simulink model "SecRwRtStFtrstHolderChk"  (R2018b)
settings: Solver=FixedStepDiscrete  StartTime=0.0  StopTime=10.0  FixedStep=0.01  RelTol=1e-3
libraries: simulink x1
settings Model: ModifiedHistory=2023/11/7Bug 555794 童锁需要停止 21-26  Creator=sn2xws  LastModifiedBy=sn2xws
settings DataIOCC: SaveFormat=StructureWithTime
settings OptimizationCC: DefaultParameterBehavior=Inlined  EnhancedBackFolding=on  PassReuseOutputArgsAs=Individual arguments  ZeroExternalMemoryAtStartup=off  ZeroInternalMemoryAtStartup=off  OptimizeBlockOrder=speed  DifferentSizesBufferReuse=on  OptimizationCustomize=off
settings DebuggingCC: ParameterTunabilityLossMsg=error
settings ModelReferenceCC: ModelReferenceNumInstancesAllowed=Single
settings SFSimCC: MATLABDynamicMemAlloc=off
settings RTWCC: SystemTargetFile=autosar.tlc  GenCodeOnly=on  TemplateMakefile=ert_default_tmf  Description=AUTOSAR  GenerateReport=on  IncludeHyperlinkInReport=on  LaunchReport=on  GenerateTraceInfo=on  GenerateTraceReport=on  GenerateTraceReportSl=on  GenerateTraceReportSf=on  GenerateTraceReportEml=on
settings CodeAppCC: ForceParamTrailComments=on  IgnoreCustomStorageClasses=off  OperatorAnnotations=on  SimulinkDataObjDesc=on  SFDataObjDesc=on  InsertBlockDesc=on
settings STFCustomTargetCC: TargetLangStandard=C99 (ISO)  MultiwordLength=256  ParMdlRefBuildCompliant=on  CompOptLevelCompliant=on  IncludeMdlTerminateFcn=off  CombineOutputUpdateFcns=on  SuppressErrorStatus=on  ERTCustomFileBanners=on  SupportNonFinite=off  SupportComplex=off  SupportContinuousTime=off  SupportNonInlinedSFcns=off  RemoveResetFunc=on  MATLABClassNameForMDSCustomization=Simulink.SoftwareTarget.ERTCustomization  AutosarCompliant=on  UseToolchainInfoCompliant=on  LookupTableObjectStructAxisOrder=2,1,3,4,...  LUTObjectStructOrderEvenSpacing=Size,Table,Breakpoints  SystemTargetFile=autosar.tlc
settings ERTTargetCC: TargetLangStandard=C99 (ISO)  ConcurrentExecutionCompliant=off  IncludeMdlTerminateFcn=off  SuppressErrorStatus=on  SupportNonFinite=off  SupportComplex=off  ModelStepFunctionPrototypeControlCompliant=off  CPPClassGenCompliant=off  AutosarCompliant=on  LookupTableObjectStructAxisOrder=2,1,3,4,...  LUTObjectStructOrderEvenSpacing=Size,Table,Breakpoints  InlinedParameterPlacement=NonHierarchical  ERTCustomFileTemplate=example_file_process.tlc  ERTFilePackagingFormat=Compact

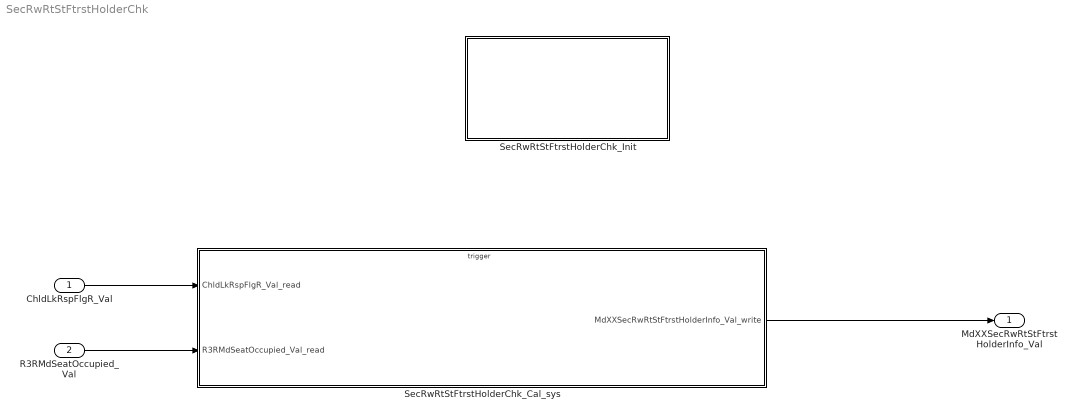
== system SecRwRtStFtrstHolderChk ==
  ChldLkRspFlgR_Val : Inport  OutDataTypeStr=boolean  PortDimensions=1
  R3RMdSeatOccupied_Val : Inport  Port=2  OutDataTypeStr=boolean  PortDimensions=1
  SecRwRtStFtrstHolderChk_Cal_sys : Subsystem
  SecRwRtStFtrstHolderChk_Init : Subsystem
  MdXXSecRwRtStFtrstHolderInfo_Val : Outport  OutDataTypeStr=uint32  PortDimensions=1
  wires:
  ChldLkRspFlgR_Val/1 -> SecRwRtStFtrstHolderChk_Cal_sys/1(ChldLkRspFlgR_Val_read)
  R3RMdSeatOccupied_Val/1 -> SecRwRtStFtrstHolderChk_Cal_sys/2(R3RMdSeatOccupied_Val_read)
  SecRwRtStFtrstHolderChk_Cal_sys/1(MdXXSecRwRtStFtrstHolderInfo_Val_write) -> MdXXSecRwRtStFtrstHolderInfo_Val/1

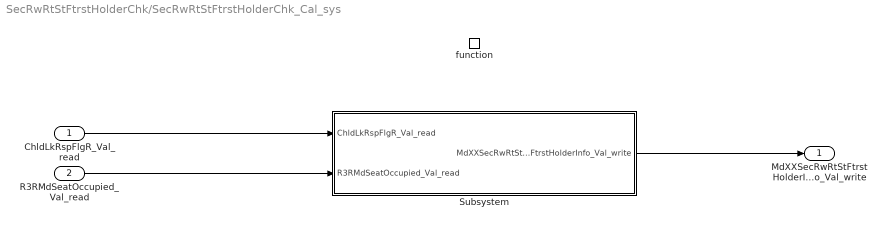
== system SecRwRtStFtrstHolderChk/SecRwRtStFtrstHolderChk_Cal_sys ==
  ChldLkRspFlgR_Val_read : Inport
  R3RMdSeatOccupied_Val_read : Inport  Port=2
  function : TriggerPort  TriggerType=function-call  IsSimulinkFunction=on  FunctionName=SecRwRtStFtrstHolderChk_Cal  VariantControl=(inherit)
  Subsystem : Subsystem
  MdXXSecRwRtStFtrstHolderInfo_Val_write : Outport
      settings: EnsureOutportIsVirtual=on
  wires:
  Subsystem/1(MdXXSecRwRtStFtrstHolderInfo_Val_write) -> MdXXSecRwRtStFtrstHolderInfo_Val_write/1
  ChldLkRspFlgR_Val_read/1 -> Subsystem/1(ChldLkRspFlgR_Val_read)
  R3RMdSeatOccupied_Val_read/1 -> Subsystem/2(R3RMdSeatOccupied_Val_read)

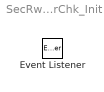
== system SecRwRtStFtrstHolderChk/SecRwRtStFtrstHolderChk_Init ==
  Event Listener : EventListener  EventName=reset

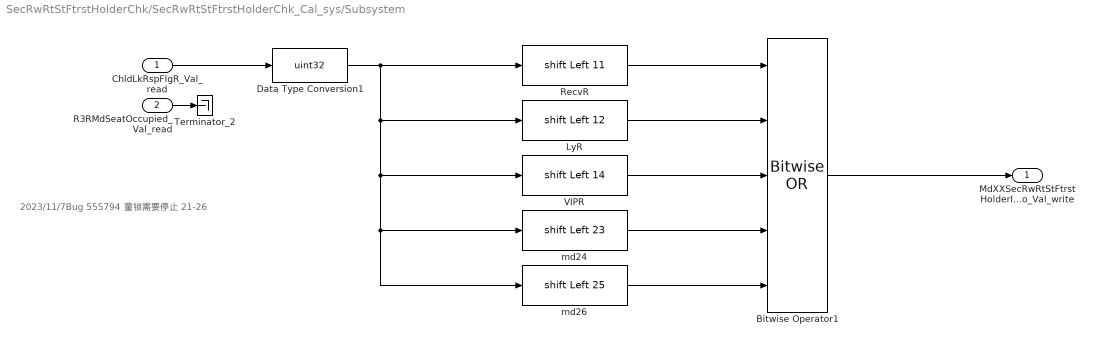
== system SecRwRtStFtrstHolderChk/SecRwRtStFtrstHolderChk_Cal_sys/Subsystem ==
  note: 2023/11/7Bug 555794 童锁需要停止 21-26
  ChldLkRspFlgR_Val_read : Inport
  R3RMdSeatOccupied_Val_read : Inport  Port=2
  Bitwise Operator1 : simulink/Logic and Bit Operations/Bitwise Operator  logicop=OR  UseBitMask=off  NumInputPorts=5  BitMask=bin2dec('11011001')  BitMaskRealWorld=Stored Integer
  Data Type Conversion1 : DataTypeConversion  OutDataTypeStr=uint32
  LyR : ArithShift  BitShiftNumber=12  BitShiftDirection=Left
  RecvR : ArithShift  BitShiftNumber=11  BitShiftDirection=Left
  Terminator_2 : Terminator
  VIPR : ArithShift  BitShiftNumber=14  BitShiftDirection=Left
  md24 : ArithShift  BitShiftNumber=23  BitShiftDirection=Left
  md26 : ArithShift  BitShiftNumber=25  BitShiftDirection=Left
  MdXXSecRwRtStFtrstHolderInfo_Val_write : Outport
      settings: EnsureOutportIsVirtual=on
  wires:
  Bitwise Operator1/1 -> MdXXSecRwRtStFtrstHolderInfo_Val_write/1
  R3RMdSeatOccupied_Val_read/1 -> Terminator_2/1
  VIPR/1 -> Bitwise Operator1/3
  ChldLkRspFlgR_Val_read/1 -> Data Type Conversion1/1
  Data Type Conversion1/1 -> RecvR/1, md26/1, md24/1, VIPR/1, LyR/1
  LyR/1 -> Bitwise Operator1/2
  RecvR/1 -> Bitwise Operator1/1
  md24/1 -> Bitwise Operator1/4
  md26/1 -> Bitwise Operator1/5
